simulink model "Antriebsmotor_V2"  (R2024a)
settings: Solver=VariableStepAuto  StartTime=0.0  StopTime=10.0  RelTol=1e-3
PreLoadFcn:
  | run('Parameter.m')
values from neighbouring files (symbols this model uses):
  AA = [-(motordamping/motorinertia) motortorquekoef/motorinertia -(1/motorinertia); -motorBackEMFkoef/motorinductivity -motorresistance/motorinductivity 0; 0 0 0 ]    [Parameter.m]
  BB = [0;1/motorinductivity;0]    [Parameter.m]
  CCT = [0 0 1]    [Parameter.m]
settings Model: Creator=jakob  LastModifiedBy=jakob

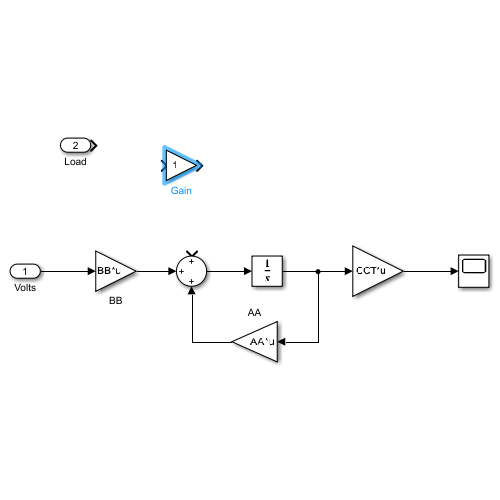
[thumbnail: Simulink's stored preview of the top-level diagram]
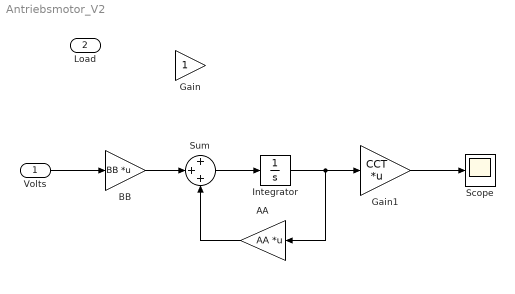
== system Antriebsmotor_V2 ==
  Volts : Inport
  Load : Inport  Port=2
  AA : Gain  Gain=AA  Multiplication=Matrix(K*u)
  BB : Gain  Gain=BB  Multiplication=Matrix(K*u)
  Gain : Gain
  Gain1 : Gain  Gain=CCT  Multiplication=Matrix(K*u)
  Integrator : Integrator
  Scope : Scope
  Sum : Sum  Inputs=+++
  wires:
  BB/1 -> Sum/2
  Sum/1 -> Integrator/1
  Integrator/1 -> AA/1, Gain1/1
  AA/1 -> Sum/3
  Gain1/1 -> Scope/1
  Volts/1 -> BB/1
